simulink model "sim_long_acc"  (R2024b)
settings: Solver=ode4  StartTime=0.0  StopTime=500  FixedStep=0.01  RelTol=1e-3
libraries: simulink x1, autolibshared x1
settings Model: Creator=fabricio  LastModifiedBy=fabricio

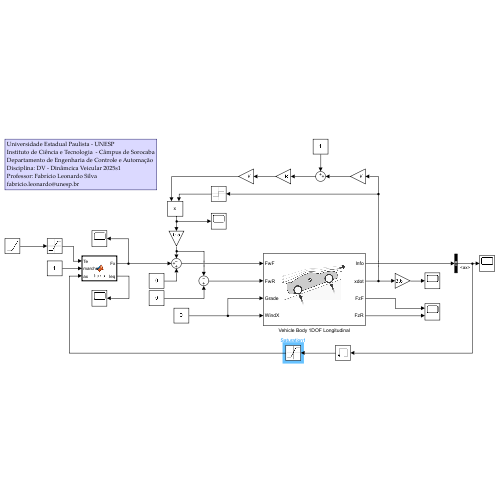
[thumbnail: Simulink's stored preview of the top-level diagram]
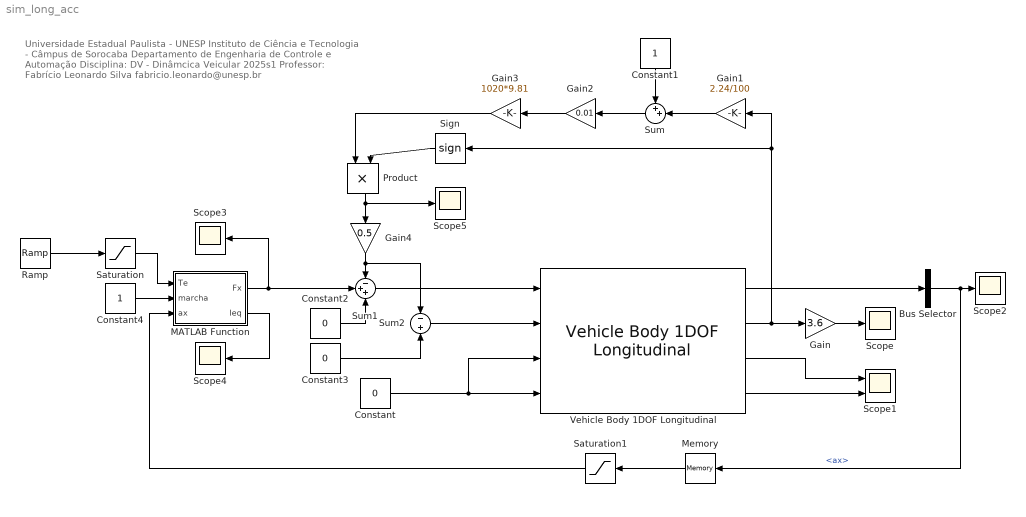
== system sim_long_acc ==
  note: Universidade Estadual Paulista - UNESP
      | Instituto de Ciência e Tecnologia - Câmpus de Sorocaba
      | Departamento de Engenharia de Controle e Automação
      | Disciplina: DV - Dinâmcica Veicular 2025s1
      | Professor: Fabrício Leonardo Silva
      | fabricio.leonardo@unesp.br
  Bus Selector : BusSelector  OutputSignals=BdyFrm.Cg.Acc.ax
  Constant : Constant  Value=0
  Constant1 : Constant
  Constant2 : Constant  Value=0
  Constant3 : Constant  Value=0
  Constant4 : Constant
  Gain : Gain  Gain=3.6
  Gain1 : Gain  Gain=2.24/100
  Gain2 : Gain  Gain=0.01
  Gain3 : Gain  Gain=1020*9.81
  Gain4 : Gain  Gain=0.5
  MATLAB Function : MATLAB Function  TreatAsAtomicUnit=on
  Memory : Memory
  Product : Product
  Ramp : simulink/Sources/Ramp  slope=5  start=0  InitialOutput=0
  Saturation : Saturate  UpperLimit=100
  Saturation1 : Saturate  UpperLimit=100  LowerLimit=0
  Scope{,2..5} (5 alike) : Scope
  Scope1 : Scope  NumInputPorts=2
  Sign : Signum
  Sum : Sum  Inputs=++|
  Sum1 : Sum  Inputs=-++
  Sum2 : Sum  Inputs=-|+
  Vehicle Body 1DOF Longitudinal : autolibshared/Vehicle Body 1DOF Longitudinal  VariantControl=SL  extFMode=off  extMMode=off  extTamb=off  wind3D=off  aMode=1  NF=2  NR=2  m=1020  a=1.4  b=1.8  h=.35  Cd=.33  Cl=0  Cpm=0  Af=2.04  x_o=0  xdot_o=0  Pabs=101325  T=273  g=9.81
      settings: LibrarySourceBlock=autolibvehdynlong/Vehicle Body 1DOF Longitudinal
  wires:
  Constant/1 -> Vehicle Body 1DOF Longitudinal/3, Vehicle Body 1DOF Longitudinal/4
  Vehicle Body 1DOF Longitudinal/2 -> Gain1/1, Sign/1, Gain/1
  Gain/1 -> Scope/1
  Gain1/1 -> Sum/2
  Sum/1 -> Gain2/1
  Constant1/1 -> Sum/1
  Gain2/1 -> Gain3/1
  Vehicle Body 1DOF Longitudinal/3 -> Scope1/1
  Vehicle Body 1DOF Longitudinal/4 -> Scope1/2
  Vehicle Body 1DOF Longitudinal/1 -> Bus Selector/1
  Bus Selector/1 -> Memory/1, Scope2/1  "<ax>"
  Sum1/1 -> Vehicle Body 1DOF Longitudinal/1
  Sign/1 -> Product/2
  Gain3/1 -> Product/1
  Product/1 -> Gain4/1, Scope5/1
  Sum2/1 -> Vehicle Body 1DOF Longitudinal/2
  Gain4/1 -> Sum2/1, Sum1/1
  Constant2/1 -> Sum1/3
  Constant3/1 -> Sum2/2
  Constant4/1 -> MATLAB Function/2(marcha)
  Saturation/1 -> MATLAB Function/1(Te)
  Ramp/1 -> Saturation/1
  MATLAB Function/2(Ieq) -> Scope4/1
  MATLAB Function/1(Fx) -> Scope3/1, Sum1/2
  Memory/1 -> Saturation1/1
  Saturation1/1 -> MATLAB Function/3(ax)

== matlab function sim_long_acc/MATLAB Function ==
  data: Te input; marcha input; Fx output; ax input; Ieq output
function [Fx,Ieq] = trans(Te,marcha,ax)

% --------------------- Motor de combustão interna -----------------------
Ie = 0.125;         % Inercia do motor/volante

% ------------------------ Sistema de Transmissão -------------------------
nt = [3.750 2.235 1.518 1.132 0.820]; % Relações de transmissão da caixa de engrenagens
it = [0.128 0.100 0.062 0.028 0.010]; % Inercia da transmissão [kg/m^2]
Nd = 2.950;         % Relação de transmissão do diferencial
Id = 0.065;          % Inercia do diferencial [kgm2]
ntd = 0.91;          % Eficiência total da transmisão

% ----------------------------- Raio do pneu ------------------------------
Rp = 0.307;         % Raio dinâmico\efetivo do pneu [m]
Iw = 0.860;          % Inercia de cada roda [kgm2]


Ntd = nt(marcha)*Nd;    % Redução total da transmissão
It = it(marcha);               % Inercia da transmissão para a marcha atual

Fx = (Te*Ntd*ntd)/Rp - ( (Ie+It)*Ntd^2 +Id*Nd^2 +2*Iw ) * (ax/(Rp^2));
if Fx<101
    Fx = 0;
end
Ieq = ( (Ie+It)*Ntd^2 +Id*Nd^2 +2*Iw ) * (ax/(Rp^2));
